simulink model "PC1"  (R2016b)
settings: Solver=VariableStepAuto  StartTime=0.0  StopTime=10  MaxStep=0.01  RelTol=1e-3
libraries: simulink x1
settings Model: Creator=BOUDOT  LastModifiedBy=BOUDOT

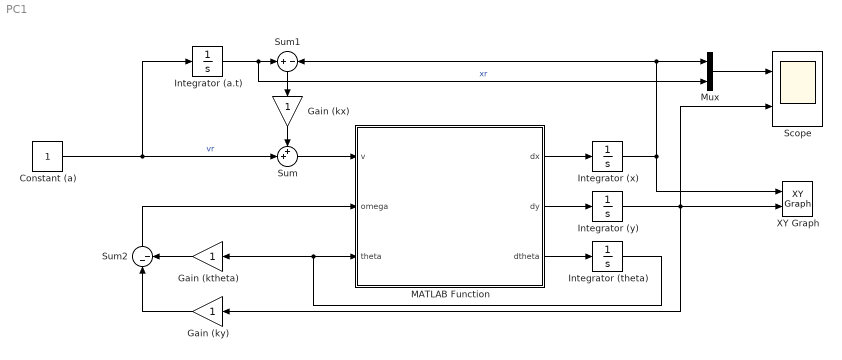
== system PC1 ==
  Constant (a) : Constant
  Gain (ktheta) : Gain
  Gain (kx) : Gain
  Gain (ky) : Gain
  Integrator (a.t) : Integrator
  Integrator (theta) : Integrator  InitialCondition=0.2
  Integrator (x) : Integrator  InitialCondition=-1
  Integrator (y) : Integrator  InitialCondition=1
  MATLAB Function : MATLAB Function  TreatAsAtomicUnit=on
  Mux : Mux  Inputs=2
  Scope : Scope  NumInputPorts=2
  Sum : Sum  Inputs=++|
  Sum1 : Sum  Inputs=+|-
  Sum2 : Sum  Inputs=|--
  XY Graph : simulink/Sinks/XY Graph  xmin=-5  xmax=15  ymin=-10  ymax=10  st=-1
  wires:
  MATLAB Function/3(dtheta) -> Integrator (theta)/1
  MATLAB Function/2(dy) -> Integrator (y)/1
  MATLAB Function/1(dx) -> Integrator (x)/1
  Integrator (theta)/1 -> MATLAB Function/3(theta), Gain (ktheta)/1
  Constant (a)/1 -> Integrator (a.t)/1, Sum/2  "vr"
  Sum/1 -> MATLAB Function/1(v)
  Integrator (a.t)/1 -> Mux/2, Sum1/1  "xr"
  Sum1/1 -> Gain (kx)/1
  Integrator (x)/1 -> Mux/1, Sum1/2, XY Graph/1
  Gain (kx)/1 -> Sum/1
  Integrator (y)/1 -> Gain (ky)/1, XY Graph/2, Scope/2
  Sum2/1 -> MATLAB Function/2(omega)
  Gain (ktheta)/1 -> Sum2/2
  Gain (ky)/1 -> Sum2/1
  Mux/1 -> Scope/1

== matlab function PC1/MATLAB Function ==
  data: v input; dx output; omega input; theta input; dy output; dtheta output
function [dx, dy, dtheta] = chariot(v, omega, theta)

dx = v*cos(theta);
dy = v*sin(theta);
dtheta = omega;
